simulink model "MBD_week2_4"  (R2020b)
settings: Solver=VariableStepAuto  StartTime=0.0  StopTime=0.2  RelTol=1e-3
model workspace (MAT data in the model file):
  J = Simulink.Parameter
  J.Value = 3.2284e-06
  J.DataType = 'auto'
  J.Dimensions = [1 1]
  Ke = Simulink.Parameter
  Ke.Value = 0.0274
  Ke.DataType = 'auto'
  Ke.Dimensions = [1 1]
  Kt = Simulink.Parameter
  Kt.Value = 0.0274
  Kt.DataType = 'auto'
  Kt.Dimensions = [1 1]
  L = Simulink.Parameter
  L.Value = 2.75e-06
  L.DataType = 'auto'
  L.Dimensions = [1 1]
  R = Simulink.Parameter
  R.Value = 4
  R.DataType = 'auto'
  R.Dimensions = [1 1]
  Ts = Simulink.Parameter
  Ts.Value = 0.01
  Ts.DataType = 'auto'
  Ts.Dimensions = [1 1]
  b = Simulink.Parameter
  b.Value = 3.5077e-06
  b.DataType = 'auto'
  b.Dimensions = [1 1]
  kd = Simulink.Parameter
  kd.Value = 50
  kd.DataType = 'auto'
  kd.Dimensions = [1 1]
  ki = Simulink.Parameter
  ki.Value = 22000
  ki.DataType = 'auto'
  ki.Dimensions = [1 1]
  kp = Simulink.Parameter
  kp.Value = 22000
  kp.DataType = 'auto'
  kp.Dimensions = [1 1]
settings Model: Creator=varunraj  LastModifiedBy=varunraj

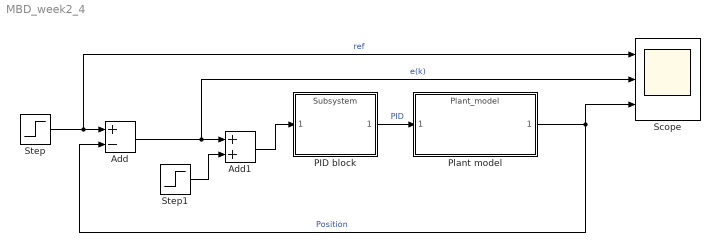
== system MBD_week2_4 ==
  Add : Sum  Inputs=+-
  Add1 : Sum
  PID block : ModelReference  ModelNameDialog=Subsystem  SimulationMode=Normal  ModelReferenceVersion=1.3
  Plant model : ModelReference  ModelNameDialog=Plant_model  SimulationMode=Normal  ModelReferenceVersion=1.3
  Scope : Scope  NumInputPorts=3
  Step : Step  Time=0.01  SampleTime=0
  Step1 : Step  Time=0.01  After=0.1  SampleTime=0
  wires:
  Add/1 -> Scope/2, Add1/1  "e(k)"
  Add1/1 -> PID block/1
  Step/1 -> Scope/1, Add/1  "ref"
  Step1/1 -> Add1/2
  PID block/1 -> Plant model/1  "PID"
  Plant model/1 -> Add/2, Scope/3  "Position"
